simulink subsystem "FromFMtoOmega2"  (R2023a)
settings: Solver=VariableStepAuto  StartTime=0.0  StopTime=10.0  RelTol=1e-3
undefined symbols (not defined in the file): HexaConstants
settings Model: Creator=Dell  LastModifiedBy=danie

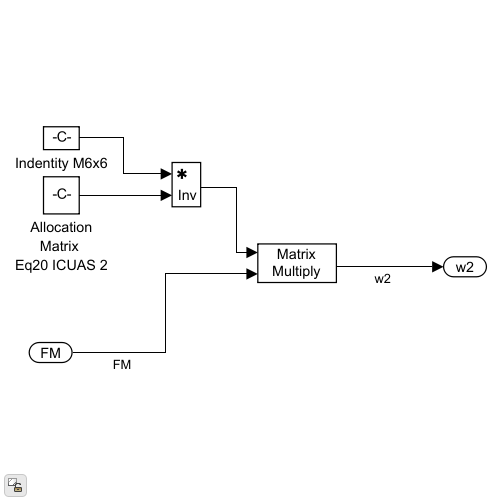
[thumbnail: Simulink's stored preview of the top-level diagram]
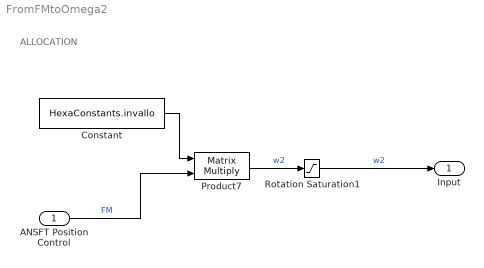
== system FromFMtoOmega2 ==
  note: ALLOCATION
  ANSFT Position Control : Inport
  Constant : Constant  Value=HexaConstants.invallo
  Product7 : Product  Multiplication=Matrix(*)
  Rotation Saturation1 : Saturate  UpperLimit=8.77e+05  LowerLimit=0
  Input : Outport
  wires:
  ANSFT Position Control/1 -> Product7/2  "FM"
  Constant/1 -> Product7/1
  Product7/1 -> Rotation Saturation1/1  "w2"
  Rotation Saturation1/1 -> Input/1  "w2"
